simulink model "new_pedal_script"  (R2021a)
settings: Solver=VariableStepAuto  StartTime=0.0  StopTime=10.0  RelTol=1e-3
PreLoadFcn:
  | data
StopFcn:
  | drawing
settings Model: Creator=Beshary  LastModifiedBy=Beshary

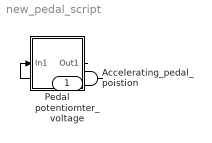
== system new_pedal_script ==
  Accelerating_pedal_poistion : Inport
  Pedal : Subsystem
  potentiomter_voltage : Outport
  wires:
  Accelerating_pedal_poistion/1 -> Pedal/1(In1)
  Pedal/1(Out1) -> potentiomter_voltage/1

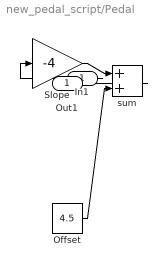
== system new_pedal_script/Pedal ==
  In1 : Inport
  Offset : Constant  Value=4.5
  Slope : Gain  Gain=-4
  sum : Sum
  Out1 : Outport
  wires:
  In1/1 -> Slope/1
  Slope/1 -> sum/1
  Offset/1 -> sum/2
  sum/1 -> Out1/1
